simulink model "JointRegulation_Yumi"  (R2024a)
settings: Solver=VariableStepDiscrete  StartTime=0.0  StopTime=10.0  MaxStep=0.004  RelTol=1e-3
undefined symbols (not defined in the file): Data, Data_SL_Info
libraries: slpidlib x14, robotlib x3
settings Model: Creator=LYA31  LastModifiedBy=LYA31

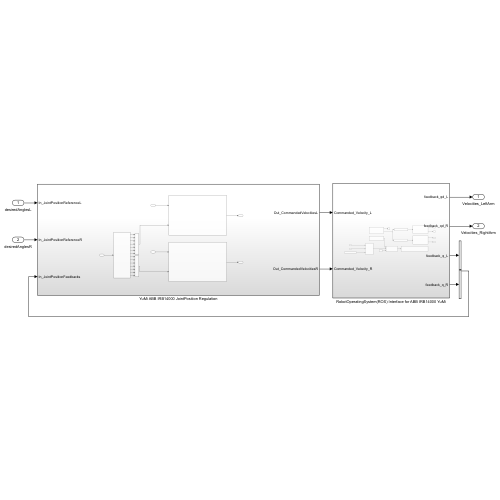
[thumbnail: Simulink's stored preview of the top-level diagram]
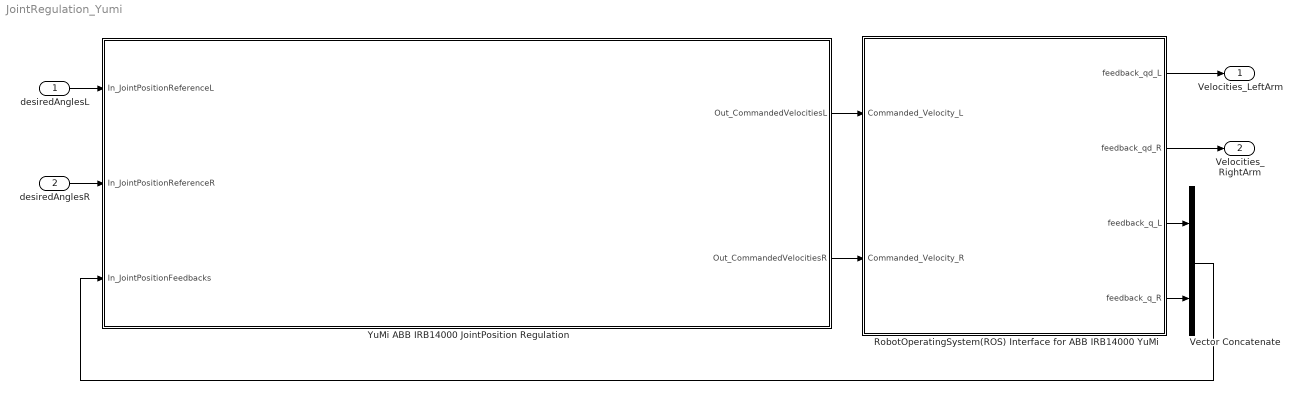
== system JointRegulation_Yumi ==
  desiredAnglesL : Inport
  desiredAnglesR : Inport  Port=2
  RobotOperatingSystem(ROS) Interface for ABB IRB14000 YuMi : Subsystem
  Vector Concatenate : Concatenate
  YuMi ABB IRB14000 JointPosition Regulation : Subsystem
  Velocities_LeftArm : Outport
  Velocities_RightArm : Outport  Port=2
  wires:
  RobotOperatingSystem(ROS) Interface for ABB IRB14000 YuMi/2(feedback_qd_R) -> Velocities_RightArm/1
  RobotOperatingSystem(ROS) Interface for ABB IRB14000 YuMi/4(feedback_q_R) -> Vector Concatenate/2
  YuMi ABB IRB14000 JointPosition Regulation/2(Out_CommandedVelocitiesR) -> RobotOperatingSystem(ROS) Interface for ABB IRB14000 YuMi/2(Commanded_Velocity_R)
  RobotOperatingSystem(ROS) Interface for ABB IRB14000 YuMi/3(feedback_q_L) -> Vector Concatenate/1
  YuMi ABB IRB14000 JointPosition Regulation/1(Out_CommandedVelocitiesL) -> RobotOperatingSystem(ROS) Interface for ABB IRB14000 YuMi/1(Commanded_Velocity_L)
  Vector Concatenate/1 -> YuMi ABB IRB14000 JointPosition Regulation/3(In_JointPositionFeedbacks)
  RobotOperatingSystem(ROS) Interface for ABB IRB14000 YuMi/1(feedback_qd_L) -> Velocities_LeftArm/1
  desiredAnglesL/1 -> YuMi ABB IRB14000 JointPosition Regulation/1(In_JointPositionReferenceL)
  desiredAnglesR/1 -> YuMi ABB IRB14000 JointPosition Regulation/2(In_JointPositionReferenceR)

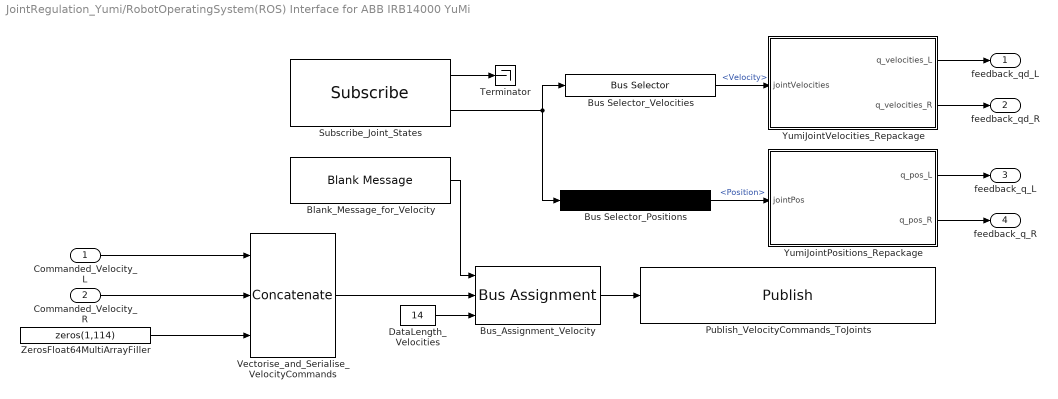
== system JointRegulation_Yumi/RobotOperatingSystem(ROS) Interface for ABB IRB14000 YuMi ==
  Commanded_Velocity_L : Inport
  Commanded_Velocity_R : Inport  Port=2
  Blank_Message_for_Velocity : robotlib/Blank Message  messageClass=Message  entityType=std_msgs/Float64MultiArray  messageType=std_msgs/Float64MultiArray  SampleTime=inf  legacyBusStruct=off
  Bus Selector_Positions : BusSelector  OutputSignals=Position
  Bus Selector_Velocities : BusSelector  OutputSignals=Velocity
  Bus_Assignment_Velocity : BusAssignment  AssignedSignals=Data,Data_SL_Info.CurrentLength
  DataLength_Velocities : Constant  Value=14  OutDataTypeStr=uint32  SampleTime=0.004
  Publish_VelocityCommands_ToJoints : robotlib/Publish  topicSource=Specify your own  topic=/yumi/egm/joint_group_velocity_controller/command  messageType=std_msgs/Float64MultiArray  legacyBusStruct=off  messageQueueLength=1
  Subscribe_Joint_States : robotlib/Subscribe  topicSource=Select from ROS network  topic=/yumi/egm/joint_states  messageType=sensor_msgs/JointState  SampleTime=-1  legacyBusStruct=off  messageQueueLength=1
  Terminator : Terminator
  Vectorise_and_Serialise_VelocityCommands : Concatenate  NumInputs=3
  YumiJointPositions_Repackage : MATLAB Function  TreatAsAtomicUnit=on
  YumiJointVelocities_Repackage : MATLAB Function  TreatAsAtomicUnit=on
  ZerosFloat64MultiArrayFiller : Constant  Value=zeros(1,114)  OutDataTypeStr=double  LockScale=on
  feedback_qd_L : Outport
  feedback_qd_R : Outport  Port=2
  feedback_q_L : Outport  Port=3
  feedback_q_R : Outport  Port=4
  wires:
  Commanded_Velocity_R/1 -> Vectorise_and_Serialise_VelocityCommands/2
  Blank_Message_for_Velocity/1 -> Bus_Assignment_Velocity/1
  Bus Selector_Positions/1 -> YumiJointPositions_Repackage/1(jointPos)  "<Position>"
  Subscribe_Joint_States/2 -> Bus Selector_Velocities/1, Bus Selector_Positions/1
  DataLength_Velocities/1 -> Bus_Assignment_Velocity/3
  Vectorise_and_Serialise_VelocityCommands/1 -> Bus_Assignment_Velocity/2
  Commanded_Velocity_L/1 -> Vectorise_and_Serialise_VelocityCommands/1
  YumiJointPositions_Repackage/2(q_pos_R) -> feedback_q_R/1
  Bus Selector_Velocities/1 -> YumiJointVelocities_Repackage/1(jointVelocities)  "<Velocity>"
  Bus_Assignment_Velocity/1 -> Publish_VelocityCommands_ToJoints/1
  YumiJointPositions_Repackage/1(q_pos_L) -> feedback_q_L/1
  YumiJointVelocities_Repackage/2(q_velocities_R) -> feedback_qd_R/1
  YumiJointVelocities_Repackage/1(q_velocities_L) -> feedback_qd_L/1
  ZerosFloat64MultiArrayFiller/1 -> Vectorise_and_Serialise_VelocityCommands/3
  Subscribe_Joint_States/1 -> Terminator/1

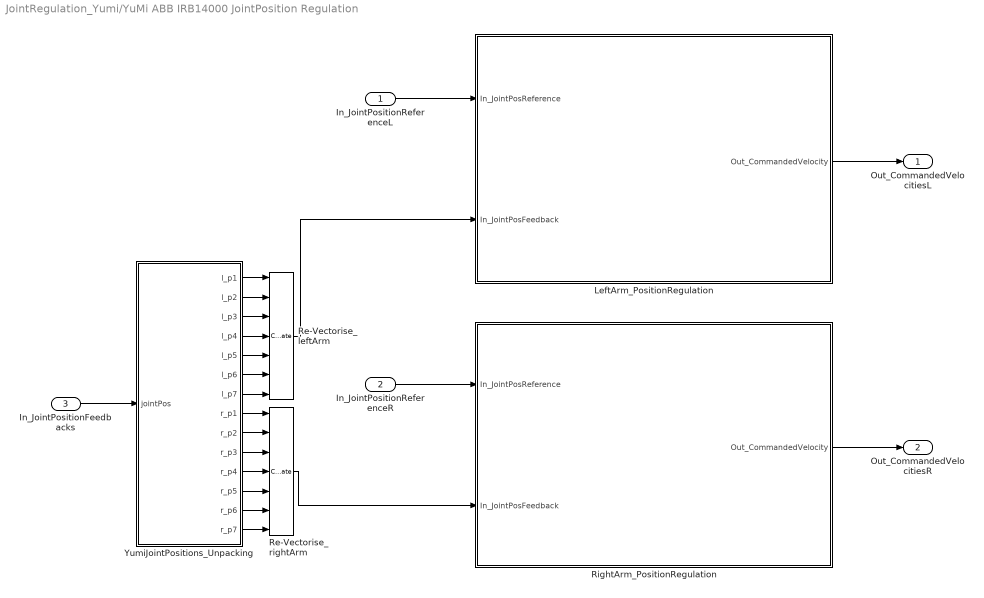
== system JointRegulation_Yumi/YuMi ABB IRB14000 JointPosition Regulation ==
  In_JointPositionReferenceL : Inport
  In_JointPositionReferenceR : Inport  Port=2
  In_JointPositionFeedbacks : Inport  Port=3
  LeftArm_PositionRegulation : Subsystem
  Re-Vectorise_leftArm : Concatenate  NumInputs=7
  Re-Vectorise_rightArm : Concatenate  NumInputs=7
  RightArm_PositionRegulation : Subsystem
  YumiJointPositions_Unpacking : MATLAB Function  TreatAsAtomicUnit=on
  Out_CommandedVelocitiesL : Outport
  Out_CommandedVelocitiesR : Outport  Port=2
  wires:
  YumiJointPositions_Unpacking/4(l_p4) -> Re-Vectorise_leftArm/4
  In_JointPositionReferenceL/1 -> LeftArm_PositionRegulation/1(In_JointPosReference)
  YumiJointPositions_Unpacking/10(r_p3) -> Re-Vectorise_rightArm/3
  Re-Vectorise_rightArm/1 -> RightArm_PositionRegulation/2(In_JointPosFeedback)
  YumiJointPositions_Unpacking/13(r_p6) -> Re-Vectorise_rightArm/6
  In_JointPositionReferenceR/1 -> RightArm_PositionRegulation/1(In_JointPosReference)
  YumiJointPositions_Unpacking/12(r_p5) -> Re-Vectorise_rightArm/5
  YumiJointPositions_Unpacking/3(l_p3) -> Re-Vectorise_leftArm/3
  YumiJointPositions_Unpacking/5(l_p5) -> Re-Vectorise_leftArm/5
  YumiJointPositions_Unpacking/8(r_p1) -> Re-Vectorise_rightArm/1
  In_JointPositionFeedbacks/1 -> YumiJointPositions_Unpacking/1(jointPos)
  YumiJointPositions_Unpacking/1(l_p1) -> Re-Vectorise_leftArm/1
  YumiJointPositions_Unpacking/6(l_p6) -> Re-Vectorise_leftArm/6
  Re-Vectorise_leftArm/1 -> LeftArm_PositionRegulation/2(In_JointPosFeedback)
  YumiJointPositions_Unpacking/11(r_p4) -> Re-Vectorise_rightArm/4
  YumiJointPositions_Unpacking/7(l_p7) -> Re-Vectorise_leftArm/7
  YumiJointPositions_Unpacking/9(r_p2) -> Re-Vectorise_rightArm/2
  YumiJointPositions_Unpacking/14(r_p7) -> Re-Vectorise_rightArm/7
  YumiJointPositions_Unpacking/2(l_p2) -> Re-Vectorise_leftArm/2
  LeftArm_PositionRegulation/1(Out_CommandedVelocity) -> Out_CommandedVelocitiesL/1
  RightArm_PositionRegulation/1(Out_CommandedVelocity) -> Out_CommandedVelocitiesR/1

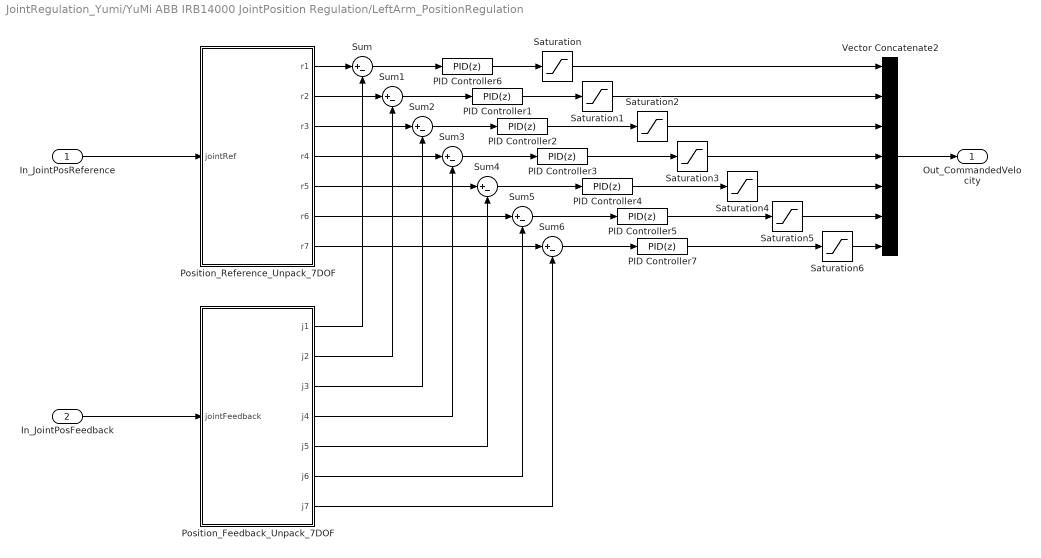
== system JointRegulation_Yumi/YuMi ABB IRB14000 JointPosition Regulation/LeftArm_PositionRegulation ==
  In_JointPosReference : Inport
  In_JointPosFeedback : Inport  Port=2
  PID Controller{1..7} (7 alike) : slpidlib/PID Controller  Controller=PID  Form=Ideal  TimeDomain=Discrete-time  UseExternalTs=off  SampleTime=-1  IntegratorMethod=Forward Euler  FilterMethod=Forward Euler  ControllerParametersSource=internal  P=9  I=0  UseKiTs=off  D=0  UseExternalDerivativeSource=off  N=100  UseFilter=on  TunerSelectOption=Transfer Function Based (PID Tuner App)  InitialConditionSource=internal  InitialConditionForIntegrator=0  InitialConditionForFilter=0  DifferentiatorICPrevScaledInput=0  ExternalReset=none  TrackingMode=off  Kt=1  LimitOutput=off  SatLimitsSource=internal  UpperSaturationLimit=inf  LowerSaturationLimit=-inf  LinearizeAsGain=on  AntiWindupMode=none  Kb=1  LimitIntegrator=off  UpperIntegratorSaturationLimit=inf  LowerIntegratorSaturationLimit=-inf  POutMin=[]  POutMax=[]  IOutMin=[]  IOutMax=[]  DOutMin=[]  DOutMax=[]  NOutMin=[]  NOutMax=[]  SumOutMin=[]  SumOutMax=[]  SaturationOutMin=[]  SaturationOutMax=[]  PParamMin=[]  PParamMax=[]  IParamMin=[]  IParamMax=[]  DParamMin=[]  DParamMax=[]  NParamMin=[]  NParamMax=[]  KbParamMin=[]  KbParamMax=[]  KtParamMin=[]  KtParamMax=[]  KbOutMin=[]  KbOutMax=[]  KtOutMin=[]  KtOutMax=[]  IntegratorOutMin=[]  IntegratorOutMax=[]  FilterOutMin=[]  FilterOutMax=[]  SumI1OutMin=[]  SumI1OutMax=[]  SumI2OutMin=[]  SumI2OutMax=[]  SumI3OutMin=[]  SumI3OutMax=[]  SumI4OutMin=[]  SumI4OutMax=[]  SumDOutMin=[]  SumDOutMax=[]  DifferentiatorOutMin=[]  DifferentiatorOutMax=[]  FilterDiffOutCoefMin=[]  FilterDiffOutCoefMax=[]  ReciprocalOutMin=[]  ReciprocalOutMax=[]  SumDenOutMin=[]  SumDenOutMax=[]  SumNumOutMin=[]  SumNumOutMax=[]  DivideOutMin=[]  DivideOutMax=[]  UdiffTsProdOutMin=[]  UdiffTsProdOutMax=[]  NTsProdOutMin=[]  NTsProdOutMax=[]  UintegralTsProdOutMin=[]  UintegralTsProdOutMax=[]  UngainTsProdOutMin=[]  UngainTsProdOutMax=[]  ClampingZeroOutDataTypeStr=Inherit: Inherit via back propagation  ClampingZeroOutMin=[]  ClampingZeroOutMax=[]  FilterDenConstantOutDataTypeStr=Inherit: Inherit via back propagation  FilterDenConstantOutMin=[]  FilterDenConstantOutMax=[]  PCopyOutDataTypeStr=Inherit: Inherit via back propagation  PCopyOutMin=[]  PCopyOutMax=[]  NCopyOutDataTypeStr=Inherit: Inherit via back propagation  NCopyOutMin=[]  NCopyOutMax=[]  IntegratorContinuousStateAttributes=''  IntegratorStateMustResolveToSignalObject=off  IntegratorRTWStateStorageClass=Auto  FilterContinuousStateAttributes=''  FilterStateMustResolveToSignalObject=off  FilterRTWStateStorageClass=Auto  ParallelPVariant=Passthrough  IdealPVariant=InternalParameters  IVariant=InternalParameters  DVariant=InternalParameters  IntegratorVariant=Discrete  SatVariant=Disabled  AWVariant=Passthrough  PCopyVariant=Disabled  TRVariant=Disabled  FdbkBlocksVariant=Forward  IdealPFdbkVariant=Disabled  SatFdbkVariant=Disabled  DerivativeFilterVariant=ForwardEulerFilter  NVariant=InternalParameters  NCopyVariant=Disabled  FilterICVariant=InternalICsFilter  IntegratorICVariant=InternalICs  ExternalResetVariant=Disabled  TRSumVariant=Passthrough  SumFdbkVariant=Disabled  SumVariant=Sum_PID  TsampFilterVariant=InternalTs  TsampNgainVariant=Passthrough  TsampIntegralVariant=Disabled_SignalSpec  ExternalSaturationOutDataTypeStr=Inherit: Same as second input  DerivativeSourceVariant=ErrorSignal
  Position_Feedback_Unpack_7DOF : MATLAB Function  TreatAsAtomicUnit=on
  Position_Reference_Unpack_7DOF : MATLAB Function  TreatAsAtomicUnit=on
  Saturation{,1..3} (4 alike) : Saturate  UpperLimit=1*pi  LowerLimit=-1*pi
  Saturation4 : Saturate  UpperLimit=(20*pi)/9  LowerLimit=-(20*pi)/9
  Saturation5 : Saturate  UpperLimit=(20*pi)/9  LowerLimit=-(20*pi)/9
  Saturation6 : Saturate  UpperLimit=(20*pi)/9  LowerLimit=-(20*pi)/9
  Sum{,1..6} (7 alike) : Sum  Inputs=|+-
  Vector Concatenate2 : Concatenate  NumInputs=7
  Out_CommandedVelocity : Outport
  wires:
  Sum2/1 -> PID Controller2/1
  Position_Reference_Unpack_7DOF/3(r3) -> Sum2/1
  Position_Reference_Unpack_7DOF/1(r1) -> Sum/1
  In_JointPosReference/1 -> Position_Reference_Unpack_7DOF/1(jointRef)
  PID Controller4/1 -> Saturation4/1
  PID Controller6/1 -> Saturation/1
  Position_Reference_Unpack_7DOF/6(r6) -> Sum5/1
  Position_Feedback_Unpack_7DOF/3(j3) -> Sum2/2
  Position_Reference_Unpack_7DOF/5(r5) -> Sum4/1
  Sum6/1 -> PID Controller7/1
  Position_Reference_Unpack_7DOF/7(r7) -> Sum6/1
  Position_Feedback_Unpack_7DOF/1(j1) -> Sum/2
  Position_Reference_Unpack_7DOF/2(r2) -> Sum1/1
  Sum4/1 -> PID Controller4/1
  Sum3/1 -> PID Controller3/1
  Position_Reference_Unpack_7DOF/4(r4) -> Sum3/1
  Position_Feedback_Unpack_7DOF/4(j4) -> Sum3/2
  Sum/1 -> PID Controller6/1
  PID Controller1/1 -> Saturation1/1
  PID Controller7/1 -> Saturation6/1
  PID Controller5/1 -> Saturation5/1
  Position_Feedback_Unpack_7DOF/7(j7) -> Sum6/2
  Sum5/1 -> PID Controller5/1
  PID Controller2/1 -> Saturation2/1
  PID Controller3/1 -> Saturation3/1
  Sum1/1 -> PID Controller1/1
  Position_Feedback_Unpack_7DOF/5(j5) -> Sum4/2
  Position_Feedback_Unpack_7DOF/2(j2) -> Sum1/2
  In_JointPosFeedback/1 -> Position_Feedback_Unpack_7DOF/1(jointFeedback)
  Vector Concatenate2/1 -> Out_CommandedVelocity/1
  Position_Feedback_Unpack_7DOF/6(j6) -> Sum5/2
  Saturation/1 -> Vector Concatenate2/1
  Saturation1/1 -> Vector Concatenate2/2
  Saturation2/1 -> Vector Concatenate2/3
  Saturation3/1 -> Vector Concatenate2/4
  Saturation4/1 -> Vector Concatenate2/5
  Saturation5/1 -> Vector Concatenate2/6
  Saturation6/1 -> Vector Concatenate2/7

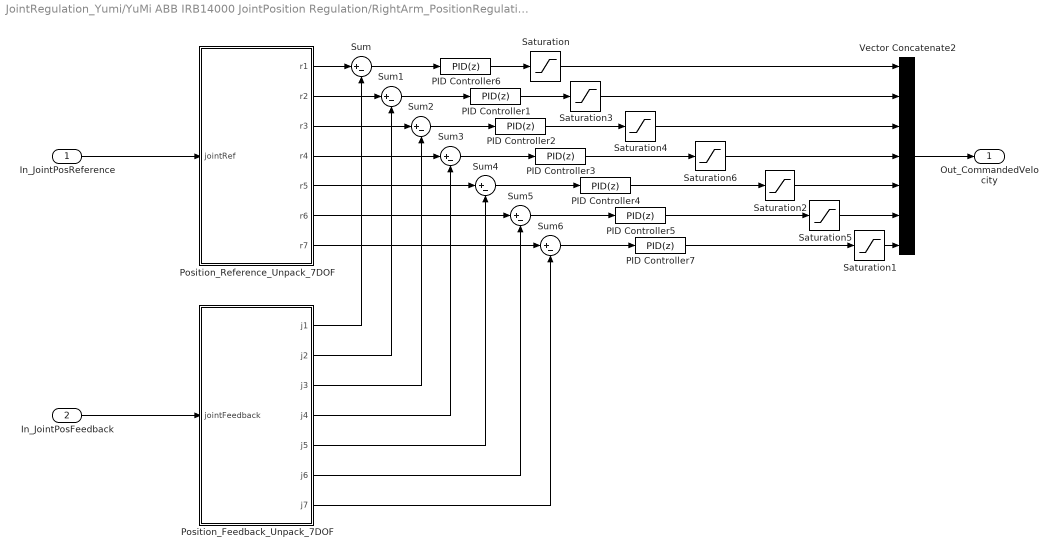
== system JointRegulation_Yumi/YuMi ABB IRB14000 JointPosition Regulation/RightArm_PositionRegulation ==
  In_JointPosReference : Inport
  In_JointPosFeedback : Inport  Port=2
  PID Controller{1..7} (7 alike) : slpidlib/PID Controller  Controller=PID  Form=Ideal  TimeDomain=Discrete-time  UseExternalTs=off  SampleTime=-1  IntegratorMethod=Forward Euler  FilterMethod=Forward Euler  ControllerParametersSource=internal  P=9  I=0  UseKiTs=off  D=0  UseExternalDerivativeSource=off  N=100  UseFilter=on  TunerSelectOption=Transfer Function Based (PID Tuner App)  InitialConditionSource=internal  InitialConditionForIntegrator=0  InitialConditionForFilter=0  DifferentiatorICPrevScaledInput=0  ExternalReset=none  TrackingMode=off  Kt=1  LimitOutput=off  SatLimitsSource=internal  UpperSaturationLimit=inf  LowerSaturationLimit=-inf  LinearizeAsGain=on  AntiWindupMode=none  Kb=1  LimitIntegrator=off  UpperIntegratorSaturationLimit=inf  LowerIntegratorSaturationLimit=-inf  POutMin=[]  POutMax=[]  IOutMin=[]  IOutMax=[]  DOutMin=[]  DOutMax=[]  NOutMin=[]  NOutMax=[]  SumOutMin=[]  SumOutMax=[]  SaturationOutMin=[]  SaturationOutMax=[]  PParamMin=[]  PParamMax=[]  IParamMin=[]  IParamMax=[]  DParamMin=[]  DParamMax=[]  NParamMin=[]  NParamMax=[]  KbParamMin=[]  KbParamMax=[]  KtParamMin=[]  KtParamMax=[]  KbOutMin=[]  KbOutMax=[]  KtOutMin=[]  KtOutMax=[]  IntegratorOutMin=[]  IntegratorOutMax=[]  FilterOutMin=[]  FilterOutMax=[]  SumI1OutMin=[]  SumI1OutMax=[]  SumI2OutMin=[]  SumI2OutMax=[]  SumI3OutMin=[]  SumI3OutMax=[]  SumI4OutMin=[]  SumI4OutMax=[]  SumDOutMin=[]  SumDOutMax=[]  DifferentiatorOutMin=[]  DifferentiatorOutMax=[]  FilterDiffOutCoefMin=[]  FilterDiffOutCoefMax=[]  ReciprocalOutMin=[]  ReciprocalOutMax=[]  SumDenOutMin=[]  SumDenOutMax=[]  SumNumOutMin=[]  SumNumOutMax=[]  DivideOutMin=[]  DivideOutMax=[]  UdiffTsProdOutMin=[]  UdiffTsProdOutMax=[]  NTsProdOutMin=[]  NTsProdOutMax=[]  UintegralTsProdOutMin=[]  UintegralTsProdOutMax=[]  UngainTsProdOutMin=[]  UngainTsProdOutMax=[]  ClampingZeroOutDataTypeStr=Inherit: Inherit via back propagation  ClampingZeroOutMin=[]  ClampingZeroOutMax=[]  FilterDenConstantOutDataTypeStr=Inherit: Inherit via back propagation  FilterDenConstantOutMin=[]  FilterDenConstantOutMax=[]  PCopyOutDataTypeStr=Inherit: Inherit via back propagation  PCopyOutMin=[]  PCopyOutMax=[]  NCopyOutDataTypeStr=Inherit: Inherit via back propagation  NCopyOutMin=[]  NCopyOutMax=[]  IntegratorContinuousStateAttributes=''  IntegratorStateMustResolveToSignalObject=off  IntegratorRTWStateStorageClass=Auto  FilterContinuousStateAttributes=''  FilterStateMustResolveToSignalObject=off  FilterRTWStateStorageClass=Auto  ParallelPVariant=Passthrough  IdealPVariant=InternalParameters  IVariant=InternalParameters  DVariant=InternalParameters  IntegratorVariant=Discrete  SatVariant=Disabled  AWVariant=Passthrough  PCopyVariant=Disabled  TRVariant=Disabled  FdbkBlocksVariant=Forward  IdealPFdbkVariant=Disabled  SatFdbkVariant=Disabled  DerivativeFilterVariant=ForwardEulerFilter  NVariant=InternalParameters  NCopyVariant=Disabled  FilterICVariant=InternalICsFilter  IntegratorICVariant=InternalICs  ExternalResetVariant=Disabled  TRSumVariant=Passthrough  SumFdbkVariant=Disabled  SumVariant=Sum_PID  TsampFilterVariant=InternalTs  TsampNgainVariant=Passthrough  TsampIntegralVariant=Disabled_SignalSpec  ExternalSaturationOutDataTypeStr=Inherit: Same as second input  DerivativeSourceVariant=ErrorSignal
  Position_Feedback_Unpack_7DOF : MATLAB Function  TreatAsAtomicUnit=on
  Position_Reference_Unpack_7DOF : MATLAB Function  TreatAsAtomicUnit=on
  Saturation{,3..4,6} (4 alike) : Saturate  UpperLimit=1*pi  LowerLimit=-1*pi
  Saturation1 : Saturate  UpperLimit=(20*pi)/9  LowerLimit=-(20*pi)/9
  Saturation2 : Saturate  UpperLimit=(20*pi)/9  LowerLimit=-(20*pi)/9
  Saturation5 : Saturate  UpperLimit=(20*pi)/9  LowerLimit=-(20*pi)/9
  Sum{,1..6} (7 alike) : Sum  Inputs=|+-
  Vector Concatenate2 : Concatenate  NumInputs=7
  Out_CommandedVelocity : Outport
  wires:
  Sum2/1 -> PID Controller2/1
  Position_Reference_Unpack_7DOF/3(r3) -> Sum2/1
  Position_Reference_Unpack_7DOF/1(r1) -> Sum/1
  In_JointPosReference/1 -> Position_Reference_Unpack_7DOF/1(jointRef)
  PID Controller4/1 -> Saturation2/1
  PID Controller6/1 -> Saturation/1
  Position_Reference_Unpack_7DOF/6(r6) -> Sum5/1
  Position_Feedback_Unpack_7DOF/3(j3) -> Sum2/2
  Position_Reference_Unpack_7DOF/5(r5) -> Sum4/1
  Sum6/1 -> PID Controller7/1
  Position_Reference_Unpack_7DOF/7(r7) -> Sum6/1
  Position_Feedback_Unpack_7DOF/1(j1) -> Sum/2
  Position_Reference_Unpack_7DOF/2(r2) -> Sum1/1
  Sum4/1 -> PID Controller4/1
  Sum3/1 -> PID Controller3/1
  Position_Reference_Unpack_7DOF/4(r4) -> Sum3/1
  Position_Feedback_Unpack_7DOF/4(j4) -> Sum3/2
  Sum/1 -> PID Controller6/1
  PID Controller1/1 -> Saturation3/1
  PID Controller7/1 -> Saturation1/1
  PID Controller5/1 -> Saturation5/1
  Position_Feedback_Unpack_7DOF/7(j7) -> Sum6/2
  Sum5/1 -> PID Controller5/1
  PID Controller2/1 -> Saturation4/1
  PID Controller3/1 -> Saturation6/1
  Sum1/1 -> PID Controller1/1
  Position_Feedback_Unpack_7DOF/5(j5) -> Sum4/2
  Position_Feedback_Unpack_7DOF/2(j2) -> Sum1/2
  In_JointPosFeedback/1 -> Position_Feedback_Unpack_7DOF/1(jointFeedback)
  Vector Concatenate2/1 -> Out_CommandedVelocity/1
  Position_Feedback_Unpack_7DOF/6(j6) -> Sum5/2
  Saturation1/1 -> Vector Concatenate2/7
  Saturation5/1 -> Vector Concatenate2/6
  Saturation2/1 -> Vector Concatenate2/5
  Saturation/1 -> Vector Concatenate2/1
  Saturation3/1 -> Vector Concatenate2/2
  Saturation4/1 -> Vector Concatenate2/3
  Saturation6/1 -> Vector Concatenate2/4

== matlab function JointRegulation_Yumi/RobotOperatingSystem(ROS) Interface for ABB IRB14000 YuMi/YumiJointVelocities_Repackage ==
  data: jointVelocities input; q_velocities_L output; q_velocities_R output
function [q_velocities_L, q_velocities_R]   = jointVelocities(jointVelocities)
    % Unpack each joint velocity from the vector
    q_velocities_L = jointVelocities(3:9);
    q_velocities_R = jointVelocities(12:18);
end

== matlab function JointRegulation_Yumi/YuMi ABB IRB14000 JointPosition Regulation/YumiJointPositions_Unpacking ==
  data: jointPos input; l_p1 output; l_p2 output; l_p3 output; l_p4 output; l_p5 output; l_p6 output; l_p7 output; r_p1 output; r_p2 output; r_p3 output; r_p4 output; r_p5 output; r_p6 output; r_p7 output
function [l_p1, l_p2, l_p3, l_p4, l_p5, l_p6, l_p7, r_p1, r_p2, r_p3, r_p4, r_p5, r_p6, r_p7]   = jointPositions(jointPos)
    % Unpack each joint position from the vector
    l_p1 = jointPos(1);
    l_p2 = jointPos(2);
    l_p3 = jointPos(3);
    l_p4 = jointPos(4);
    l_p5 = jointPos(5);
    l_p6 = jointPos(6);
    l_p7 = jointPos(7);
    r_p1 = jointPos(8);
    r_p2 = jointPos(9);
    r_p3 = jointPos(10);
    r_p4 = jointPos(11);
    r_p5 = jointPos(12);
    r_p6 = jointPos(13);
    r_p7 = jointPos(14);
end

== matlab function JointRegulation_Yumi/YuMi ABB IRB14000 JointPosition Regulation/LeftArm_PositionRegulation/Position_Reference_Unpack_7DOF ==
  data: jointRef input; r1 output; r2 output; r3 output; r4 output; r5 output; r6 output; r7 output
function [r1, r2, r3, r4, r5, r6, r7] = PosRef(jointRef)
    % Unpack each joint position from the vector
    r1 = jointRef(1);
    r2 = jointRef(2);
    r3 = jointRef(3);
    r4 = jointRef(4);
    r5 = jointRef(5);
    r6 = jointRef(6);
    r7 = jointRef(7);
end

== matlab function JointRegulation_Yumi/YuMi ABB IRB14000 JointPosition Regulation/LeftArm_PositionRegulation/Position_Feedback_Unpack_7DOF ==
  data: jointFeedback input; j1 output; j2 output; j3 output; j4 output; j5 output; j6 output; j7 output
function [j1, j2, j3, j4, j5, j6, j7] = PosFeedback(jointFeedback)
    % Unpack each joint position from the vector
    j1 = jointFeedback(1);
    j2 = jointFeedback(2);
    j3 = jointFeedback(3);
    j4 = jointFeedback(4);
    j5 = jointFeedback(5);
    j6 = jointFeedback(6);
    j7 = jointFeedback(7);
end

== matlab function JointRegulation_Yumi/YuMi ABB IRB14000 JointPosition Regulation/RightArm_PositionRegulation/Position_Feedback_Unpack_7DOF ==
  data: jointFeedback input; j1 output; j2 output; j3 output; j4 output; j5 output; j6 output; j7 output
function [j1, j2, j3, j4, j5, j6, j7] = PosFeedback(jointFeedback)
    % Unpack each joint position from the vector
    j1 = jointFeedback(1);
    j2 = jointFeedback(2);
    j3 = jointFeedback(3);
    j4 = jointFeedback(4);
    j5 = jointFeedback(5);
    j6 = jointFeedback(6);
    j7 = jointFeedback(7);
end

== matlab function JointRegulation_Yumi/YuMi ABB IRB14000 JointPosition Regulation/RightArm_PositionRegulation/Position_Reference_Unpack_7DOF ==
  data: jointRef input; r1 output; r2 output; r3 output; r4 output; r5 output; r6 output; r7 output
function [r1, r2, r3, r4, r5, r6, r7] = PosRef(jointRef)
    % Unpack each joint position from the vector
    r1 = jointRef(1);
    r2 = jointRef(2);
    r3 = jointRef(3);
    r4 = jointRef(4);
    r5 = jointRef(5);
    r6 = jointRef(6);
    r7 = jointRef(7);
end

== matlab function JointRegulation_Yumi/RobotOperatingSystem(ROS) Interface for ABB IRB14000 YuMi/YumiJointPositions_Repackage ==
  data: jointPos input; q_pos_L output; q_pos_R output
function [q_pos_L, q_pos_R]   = jointPositions(jointPos)
    % Unpack each joint position from the vector
    q_pos_L = jointPos(3:9);
    q_pos_R = jointPos(12:18);
end
